simulink model "c28069_SCIledBR_T"  (R2018b)
settings: Solver=ode4  StartTime=0.0  StopTime=inf  FixedStep=Ts  RelTol=1e-3
InitFcn:
  | Ts=1e-4
undefined symbols (not defined in the file): serial
libraries: instrumentlib x2
settings Model: Creator=matti  LastModifiedBy=matti
settings HardwareCC: ProdBitPerPointer=32  ProdBitPerSizeT=32  ProdBitPerPtrDiffT=32  ProdWordSize=32  ProdHWDeviceType=Intel->x86-32 (Windows32)
settings SFSimCC: SimUseLocalCustomCode=off
settings RTWCC: RTWUseLocalCustomCode=off
settings CodeAppCC: StateflowObjectComments=on
settings SimscapeCC: SimscapeNormalizeSystem=off

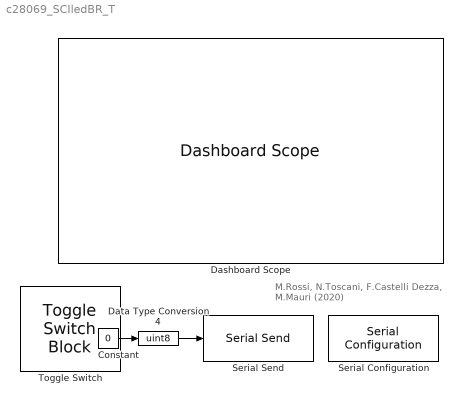
== system c28069_SCIledBR_T ==
  note: M.Rossi, N.Toscani, F.Castelli Dezza, M.Mauri (2020)
  Constant : Constant  Value=0  SampleTime=0.1
  Dashboard Scope : DashboardScope  WebBlockId=52  TimeSpan=30  Ymin=0  Ymax=2
  Data Type Conversion4 : DataTypeConversion  OutDataTypeStr=uint8
  Serial Configuration : instrumentlib/Serial Configuration  Priority=-200000  ComPortMenu=<Please select a port...>  ComPort=COM10  ObjConstructor=serial('COM10');  BaudRate=115200  DataBits=8  Parity=none  StopBits=1  FlowControl=none  Timeout=10  ByteOrder=LittleEndian
  Serial Send : instrumentlib/Serial Send  ComPortMenu=<Please select a port...>  ComPort=COM10  ObjConstructor=serial('COM10');  Terminator=<none>  EnableBlockingMode=on
  Toggle Switch : ToggleSwitchBlock  WebBlockId=94  LabelPosition=Hide
      settings: Values={{'Off', 'On'}, [0 1]}
  wires:
  Constant/1 -> Data Type Conversion4/1
  Data Type Conversion4/1 -> Serial Send/1
